simulink library "Kind"  (R2017a)
settings: Solver=VariableStepAuto  StartTime=0.0  StopTime=10.0  RelTol=1e-3
undefined symbols (not defined in the file or in its folder): contractAfterSimulation, contractBeforeSimulation, saveValidatorParameters
undefined symbols (not defined in the file): ArrowOperator, ContractAssumeBlock, ContractBlock, ContractEnsureBlock, ContractGuaranteeBlock, ContractModeBlock, ContractRequireBlock, ContractValidatorBlock
libraries: Kind x3
settings Model: Creator=mudat  LastModifiedBy=mahgoubyahia

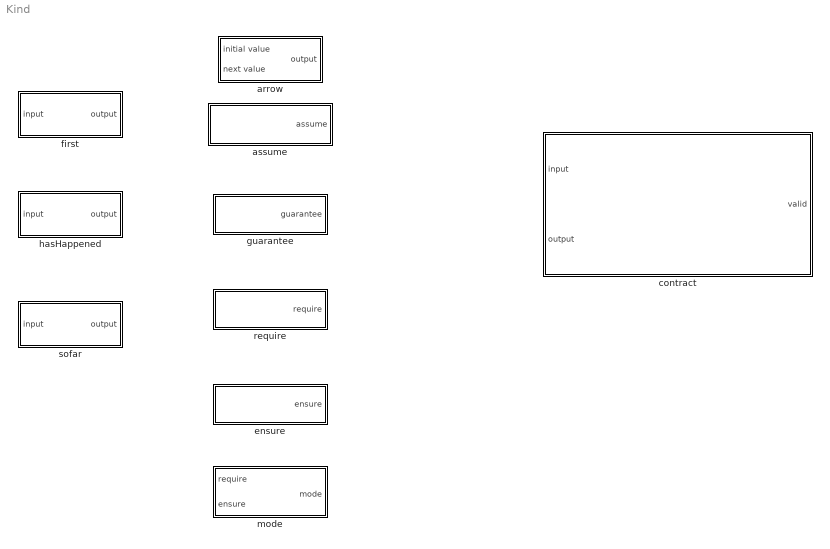
== system Kind ==
  arrow : Subsystem  mask{LustreOperatorBlock=ArrowOperator}
      mask prompts: LustreOperatorBlock "ArrowOperator"
  assume : Subsystem  mask{ContractBlockType=ContractAssumeBlock}
      mask init:
      | set_param(gcb, 'LinkStatus', 'none');
      mask DialogControl DescTextVar Prompt: Assume block
  contract : Subsystem  mask{ContractBlockType=ContractBlock}
      mask init:
      | set_param(gcb, 'LinkStatus', 'none');
      settings: CopyFcn=set_param(gcb, 'LinkStatus', 'none');
      mask DialogControl DescTextVar Prompt: Contract block
      mask Display:
      | text(0.5, 0.5, '{\bf\fontsize{20}Contract}', 'hor', 'center', 'texmode','on');
      | blocks = find_system(gcb, 'LookUnderMasks','all', 'SearchDepth',1,'BlockType','Inport');
      | for i = 1 : length(blocks)
      |     blockName = get_param(blocks(i), 'Name');
      |     [path, blockName] = fileparts(char(blockName));
      |     port_label('input', i, blockName);
      | end
      | 
      | blocks = find_system(gcb, 'LookUnderMasks','all', 'SearchDepth',1,'BlockType','Outport');
      | for i = 1 : length(blocks)
      |     blockName = get_param(blocks(i), 'Name');
      |     [path, blockName] = fileparts(char(blockName));
      |     port_label('output', i, blockName);
      | end
  ensure : Subsystem  mask{ContractBlockType=ContractEnsureBlock}
      mask init:
      | set_param(gcb, 'LinkStatus', 'none');
      mask DialogControl DescTextVar Prompt: Ensure block
  first : Subsystem
  guarantee : Subsystem  mask{ContractBlockType=ContractGuaranteeBlock}
      mask init:
      | set_param(gcb, 'LinkStatus', 'none');
      mask DialogControl DescTextVar Prompt: Guarantee block
  hasHappened : Subsystem
  mode : Subsystem  mask{ContractBlockType=ContractModeBlock}
      mask init:
      | set_param(gcb, 'LinkStatus', 'none');
      mask DialogControl DescTextVar Prompt: Mode block
  require : Subsystem  mask{ContractBlockType=ContractRequireBlock}
      mask init:
      | set_param(gcb, 'LinkStatus', 'none');
      mask DialogControl DescTextVar Prompt: Require block
  sofar : Subsystem

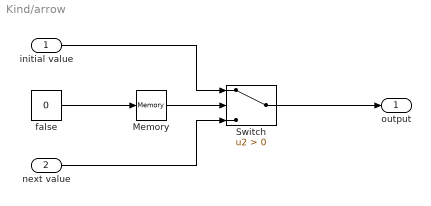
== system Kind/arrow ==
  initial value : Inport
  next value : Inport  Port=2
  Memory : Memory  X0=1
  Switch : Switch  Criteria=u2 > Threshold
  false : Constant  Value=0  OutDataTypeStr=boolean
  output : Outport
  wires:
  Switch/1 -> output/1
  next value/1 -> Switch/3
  Memory/1 -> Switch/2
  false/1 -> Memory/1
  initial value/1 -> Switch/1

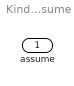
== system Kind/assume ==
  assume : Outport  OutDataTypeStr=boolean

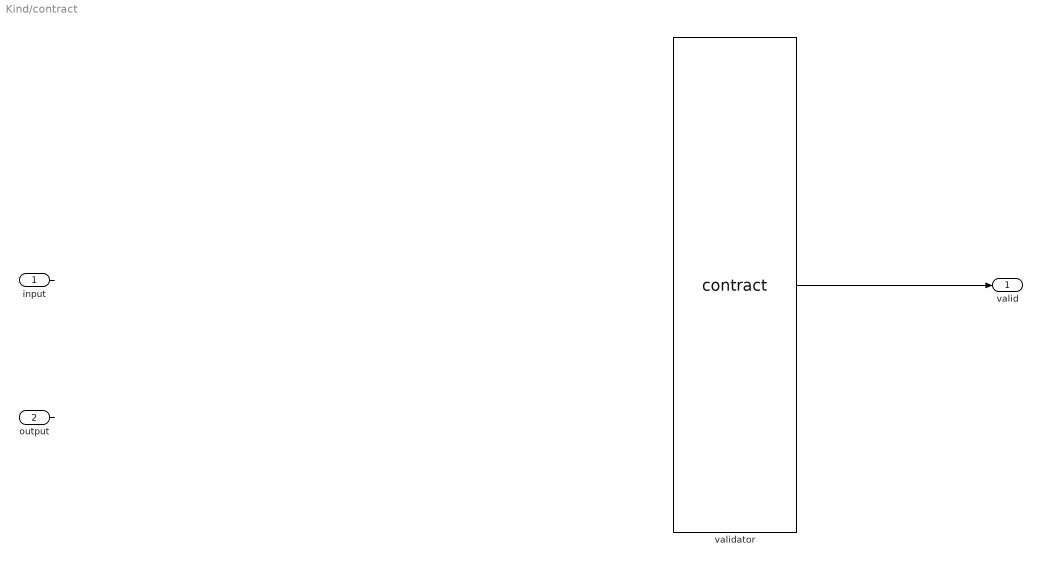
== system Kind/contract ==
  input : Inport
  output : Inport  Port=2
  validator : M-S-Function  LoadFcn=saveValidatorParameters(gcb);  InitFcn=contractBeforeSimulation();  StopFcn=contractAfterSimulation();  FunctionName=contract  mask(KindContractValidator){assumePorts=1, guaranteePorts=1, modePorts=3, ContractBlockType=ContractValidatorBlock, createInportsCheckbox=off}
      mask prompts: assumePorts "Assume ports     :"; guaranteePorts "Guarantee ports :"; modePorts "Mode ports        :"; createInportsCheckbox "Create inports and connect them automatically"
      mask init:
      | set_param(gcb,'LinkStatus','none');
      | contract_callback('inputs_callback',gcb);
      mask DialogControl DescTextVar Prompt: The validator block implements the following logic: <br> <br> <b>Sofar</b>(assume<sub>1</sub> <b>&#8743;</b> assume<sub>2</sub> <b>&#8743;</b> ... assume<sub>k</sub>) <b>&rarr;</b> (guarantee<sub>1</sub> <b>&#8743;</b> guarantee<sub>2</sub> <b>&#8743;</b> ... guarantee<sub>m</sub> <b>&#8743;</b>  mode<sub>1</sub> <b>&#8743;</b> mode<sub>2</sub> <b>&#8743;</b> ... <b>&#8743;</b> mode<sub>n</sub> )<br> where mode<sub>i</sub> = require<sub>i</sub> <b>&rarr;</b> ensure<sub>i</sub>
      mask Display:
      | port_label('input',1,'assume')
      | port_label('input',2,'guarantee')
      | port_label('input',3,'mode')
      | port_label('input',4,'mode')
      | port_label('input',5,'mode')
      | port_label('output',1,'valid')
  valid : Outport
  wires:
  validator/1 -> valid/1
  input/1 -> ?
  output/1 -> ?

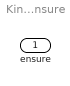
== system Kind/ensure ==
  ensure : Outport  OutDataTypeStr=boolean

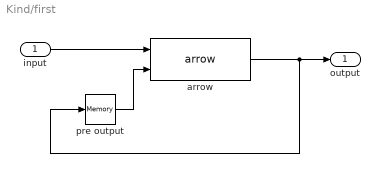
== system Kind/first ==
  input : Inport
  arrow : Kind/arrow  LustreOperatorBlock=ArrowOperator
      settings: SourceProductName=Kind lib
  pre output : Memory  X0=1
  output : Outport
  wires:
  arrow/1 -> pre output/1, output/1
  input/1 -> arrow/1
  pre output/1 -> arrow/2

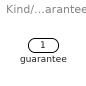
== system Kind/guarantee ==
  guarantee : Outport  OutDataTypeStr=boolean

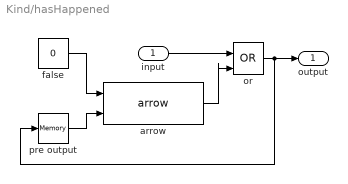
== system Kind/hasHappened ==
  input : Inport  OutDataTypeStr=boolean
  arrow : Kind/arrow  LustreOperatorBlock=ArrowOperator
      settings: SourceProductName=Kind lib
  false : Constant  Value=0  OutDataTypeStr=boolean
  or : Logic  Operator=OR  IconShape=distinctive  AllPortsSameDT=off  OutDataTypeStr=boolean
  pre output : Memory  X0=1
  output : Outport  OutDataTypeStr=boolean
  wires:
  pre output/1 -> arrow/2
  input/1 -> or/1
  false/1 -> arrow/1
  or/1 -> output/1, pre output/1
  arrow/1 -> or/2

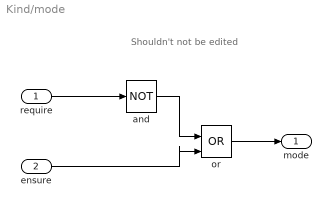
== system Kind/mode ==
  note: Shouldn't not be edited
  require : Inport  OutDataTypeStr=boolean
  ensure : Inport  Port=2  OutDataTypeStr=boolean
  and : Logic  Operator=NOT  IconShape=distinctive  AllPortsSameDT=off  OutDataTypeStr=boolean
  or : Logic  Operator=OR  IconShape=distinctive  AllPortsSameDT=off  OutDataTypeStr=boolean
  mode : Outport
  wires:
  or/1 -> mode/1
  and/1 -> or/1
  ensure/1 -> or/2
  require/1 -> and/1

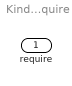
== system Kind/require ==
  require : Outport  OutDataTypeStr=boolean

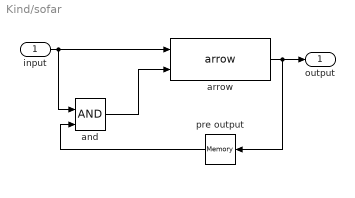
== system Kind/sofar ==
  input : Inport  OutDataTypeStr=boolean
  and : Logic  IconShape=distinctive  AllPortsSameDT=off  OutDataTypeStr=boolean
  arrow : Kind/arrow  LustreOperatorBlock=ArrowOperator
      settings: SourceProductName=Kind lib
  pre output : Memory  X0=1
  output : Outport  OutDataTypeStr=boolean
  wires:
  input/1 -> arrow/1, and/1
  arrow/1 -> pre output/1, output/1
  and/1 -> arrow/2
  pre output/1 -> and/2
